simulink model "youbot_predefinedpath_2103"  (R2025b)
settings: Solver=ode3  StartTime=0.0  StopTime=inf  FixedStep=0.01  RelTol=1e-3  EnableMultiTasking=on
values from neighbouring files (symbols this model uses):
  dt = (tf-ti)/n    (= 0.05)    [sss.m]    (also in youbotdynamiceqn.m = 0.1; youbotdynamiceqn_predefinedpath.m)
  Kdx = 1.5    [sss.m]    (also in youbotdynamiceqn_predefinedpath.m)
  Kdy = 1.5    [sss.m]    (also in youbotdynamiceqn_predefinedpath.m)
  Kdz = 0.001    [sss.m]    (also in youbotdynamiceqn_predefinedpath.m = 2.5)
  Kpx = 10    [sss.m]    (also in youbotdynamiceqn_predefinedpath.m = 1.5)
  Kpy = 10    [sss.m]    (also in youbotdynamiceqn_predefinedpath.m = 1.5)
  Kpz = 1    [sss.m]    (also in youbotdynamiceqn_predefinedpath.m = 2.5)
  M_r = [m  0  0 ... (first row only)    [sss.m]    (also in youbotdynamiceqn.m; youbotdynamiceqn_predefinedpath.m)
  M_w = diag([I_w1, I_w2, I_w3, I_w4])    [sss.m]    (also in youbotdynamiceqn.m; youbotdynamiceqn_predefinedpath.m)
  R = (1/r) * [  1, -1, -(L+l) ... (first row only)    [sss.m]    (also in youbotdynamiceqn.m; youbotdynamiceqn_predefinedpath.m)
  R_T = transpose(R)    [sss.m]    (also in youbotdynamiceqn.m; youbotdynamiceqn_predefinedpath.m)
undefined symbols (not defined in the file or in its folder): Angular, Linear
libraries: robotlib x3, robotgazebolib x1, slpidlib x1
settings Model: SimulationMode=accelerator  PacingRate=0.790000  Creator=The MathWorks, Inc.  LastModifiedBy=sinan
settings SolverCC: AlgebraicLoopSolver=TrustRegion  AutoInsertRateTranBlk=on
settings DataIOCC: LimitDataPoints=on  SaveFormat=Array  ReturnWorkspaceOutputs=off
settings OptimizationCC: ZeroExternalMemoryAtStartup=off  ZeroInternalMemoryAtStartup=off  LifeSpan=1  MaxStackSize=64
settings DebuggingCC: AlgebraicLoopMsg=none  SolverPrmCheckMsg=warning  UnconnectedInputMsg=warning  UnconnectedOutputMsg=warning  UnconnectedLineMsg=warning  SFUnexpectedBacktrackingDiag=warning  SFNoUnconditionalDefaultTransitionDiag=warning  SFExecutionAtInitializationDiag=none  ArithmeticOperatorsInVariantConditions=warning
settings HardwareCC: ProdBitPerPointer=32.0  ProdBitPerSizeT=32.0  ProdBitPerPtrDiffT=32.0  ProdLargestAtomicFloat=None  ProdIntDivRoundTo=Undefined  ProdEndianess=Unspecified  ProdWordSize=32.0  ProdHWDeviceType=Generic->Unspecified (assume 32-bit Generic)  TargetHWDeviceType=Generic->Unspecified (assume 32-bit Generic)  UseEmbeddedCoderFeatures=off
settings ModelReferenceCC: EnableRefExpFcnMdlSchedulingChecks=on  PropagateSignalLabelsOutOfModel=off
settings SFSimCC: SimUseLocalCustomCode=off  CustomCodeUndefinedFunction=UseInterfaceOnly  SimTargetLang=C++  SimDLTargetLibrary=mkl-dnn
settings RTWCC: SystemTargetFile=ert.tlc  HardwareBoard=Robot Operating System (ROS)  TLCOptions=-aInlineSetEventsForThisBaseRateFcn=TLC_FALSE -aSuppressMultiTaskScheduler=TLC_FALSE -aRateBasedStepFcn=0  TemplateMakefile=ert_default_tmf  RTWUseLocalCustomCode=off  Toolchain=Catkin  TargetLang=C++  GPUComputeCapability=3.5  Description=Embedded Coder
settings CodeAppCC: StateflowObjectComments=on
settings ERTTargetCC: InlinedParameterPlacement=Hierarchical  RootIOFormat=Structure reference  ConvertIfToSwitch=off  SuppressUnreachableDefaultCases=off  DynamicArrayContainerType=coder::array  MultiwordLength=2048.0  ERTCustomFileBanners=off  CodeInterfacePackaging=C++ class  SupportContinuousTime=on  SupportNonInlinedSFcns=on  RemoveResetFunc=off  SupportVariableSizeSignals=on  ModelStepFunctionPrototypeControlCompliant=off
settings ConfigComp: CovMetricSettings=dw  CovSaveCumulativeToWorkspaceVar=on  CovSaveSingleToWorkspaceVar=on  CovExternalEMLEnable=off  CovSFcnEnable=off
settings SimscapeCC: SimscapeLogDecimation=1  SimscapeLogDataHistory=5000

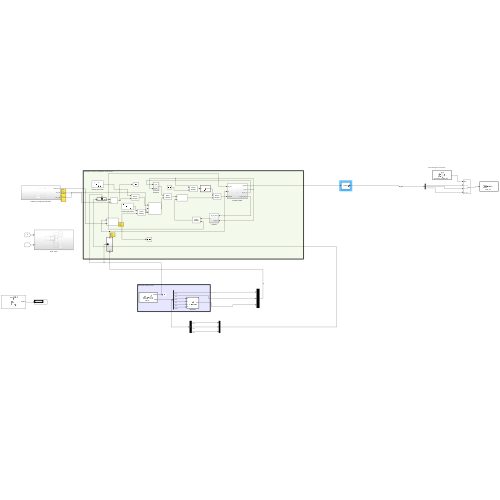
[thumbnail: Simulink's stored preview of the top-level diagram]
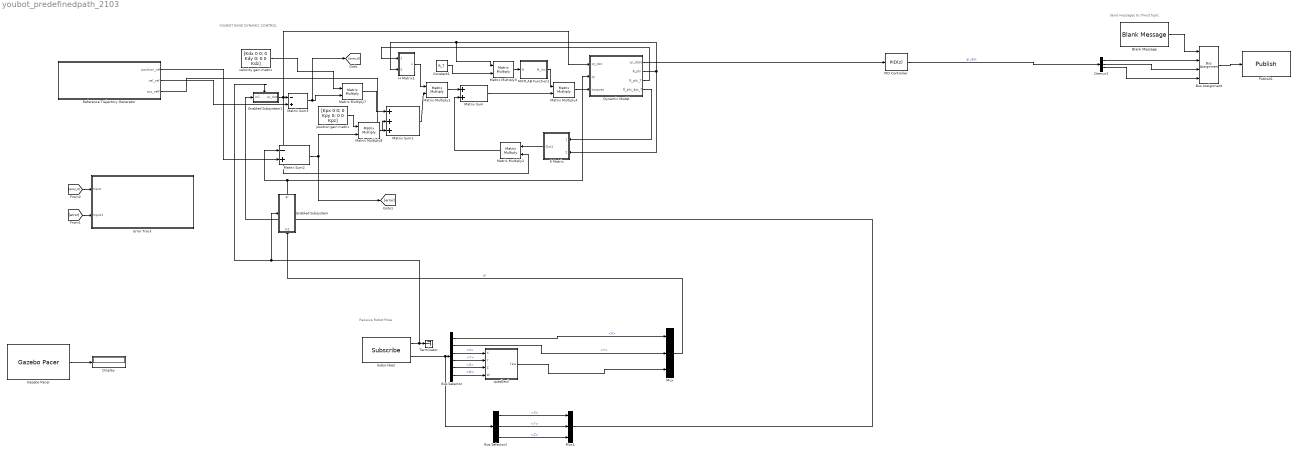
== system youbot_predefinedpath_2103 ==
  note: YOUBOT BASE DYNAMIC CONTROL
  note: Send messages to /Twist topic
  note: Receive Robot Pose
  Blank Message : robotlib/Blank Message  messageClass=Message  entityType=geometry_msgs/Twist  messageType=geometry_msgs/Twist  SampleTime=inf  legacyBusStruct=off
  Bus Assignment : BusAssignment  AssignedSignals=Linear.X,Linear.Y,Angular.Z
  Bus Selector : BusSelector  OutputSignals=Pose.Pose.Position.X,Pose.Pose.Position.Y,Pose.Pose.Orientation.X,Pose.Pose.Orientation.Y,Pose.Pose.Orientation.Z,Pose.Pose.Orientation.W
  Bus Selector1 : BusSelector  OutputSignals=Twist.Twist.Linear.X,Twist.Twist.Linear.Y,Twist.Twist.Angular.Z
  Constant1 : Constant  Value=R_T
  Demux1 : Demux  Outputs=3
  Display : Display
  Dynamic Model : Subsystem
  Enabled Subsystem : Subsystem  TreatAsAtomicUnit=on
  Enabled Subsystem1 : Subsystem  TreatAsAtomicUnit=on
  Error Track : Subsystem
  Gazebo Pacer : robotgazebolib/Gazebo Pacer  ResetBehavior=Reset Gazebo simulation time  SampleTime=0.001
  H Matrix1 : Subsystem
  K Matrix : Subsystem
  MATLAB Function1 : MATLAB Function  TreatAsAtomicUnit=on
  Matrix Sum : Sum
  Matrix Sum1 : Sum  Inputs=+++
  Matrix Sum2 : Sum  Inputs=-+
  Matrix Sum3 : Sum  Inputs=-+
  Matrix Multiply1 : Product  Multiplication=Matrix(*)  SampleTime=dt
  Matrix Multiply{2..4,7..8} (5 alike) : Product  Multiplication=Matrix(*)
  Mux : Mux  Inputs=3
  Mux1 : Mux  Inputs=3
  PID Controller : slpidlib/PID Controller  Controller=PID  Form=Parallel  TimeDomain=Discrete-time  UseExternalTs=off  SampleTime=-1  IntegratorMethod=Forward Euler  FilterMethod=Forward Euler  ControllerParametersSource=internal  P=1  I=0  UseKiTs=off  D=0  UseExternalDerivativeSource=off  N=100  UseFilter=on  TunerSelectOption=Transfer Function Based (PID Tuner App)  InitialConditionSource=internal  InitialConditionForIntegrator=0  InitialConditionForFilter=0  DifferentiatorICPrevScaledInput=0  ExternalReset=none  TrackingMode=off  Kt=1  LimitOutput=on  SatLimitsSource=internal  UpperSaturationLimit=1.5  LowerSaturationLimit=-1.5  LinearizeAsGain=on  AntiWindupMode=clamping  Kb=1  LimitIntegrator=off  UpperIntegratorSaturationLimit=inf  LowerIntegratorSaturationLimit=-inf  POutMin=[]  POutMax=[]  IOutMin=[]  IOutMax=[]  DOutMin=[]  DOutMax=[]  NOutMin=[]  NOutMax=[]  SumOutMin=[]  SumOutMax=[]  SaturationOutMin=[]  SaturationOutMax=[]  PParamMin=[]  PParamMax=[]  IParamMin=[]  IParamMax=[]  DParamMin=[]  DParamMax=[]  NParamMin=[]  NParamMax=[]  KbParamMin=[]  KbParamMax=[]  KtParamMin=[]  KtParamMax=[]  KbOutMin=[]  KbOutMax=[]  KtOutMin=[]  KtOutMax=[]  IntegratorOutMin=[]  IntegratorOutMax=[]  FilterOutMin=[]  FilterOutMax=[]  SumI1OutMin=[]  SumI1OutMax=[]  SumI2OutMin=[]  SumI2OutMax=[]  SumI3OutMin=[]  SumI3OutMax=[]  SumI4OutMin=[]  SumI4OutMax=[]  SumDOutMin=[]  SumDOutMax=[]  DifferentiatorOutMin=[]  DifferentiatorOutMax=[]  FilterDiffOutCoefMin=[]  FilterDiffOutCoefMax=[]  ReciprocalOutMin=[]  ReciprocalOutMax=[]  SumDenOutMin=[]  SumDenOutMax=[]  SumNumOutMin=[]  SumNumOutMax=[]  DivideOutMin=[]  DivideOutMax=[]  UdiffTsProdOutMin=[]  UdiffTsProdOutMax=[]  NTsProdOutMin=[]  NTsProdOutMax=[]  UintegralTsProdOutMin=[]  UintegralTsProdOutMax=[]  UngainTsProdOutMin=[]  UngainTsProdOutMax=[]  ClampingZeroOutDataTypeStr=Inherit: Inherit via back propagation  ClampingZeroOutMin=[]  ClampingZeroOutMax=[]  FilterDenConstantOutDataTypeStr=Inherit: Inherit via back propagation  FilterDenConstantOutMin=[]  FilterDenConstantOutMax=[]  PCopyOutDataTypeStr=Inherit: Inherit via back propagation  PCopyOutMin=[]  PCopyOutMax=[]  NCopyOutDataTypeStr=Inherit: Inherit via back propagation  NCopyOutMin=[]  NCopyOutMax=[]  IntegratorContinuousStateAttributes=''  IntegratorStateMustResolveToSignalObject=off  IntegratorRTWStateStorageClass=Auto  FilterContinuousStateAttributes=''  FilterStateMustResolveToSignalObject=off  FilterRTWStateStorageClass=Auto  ParallelPVariant=InternalParameters  IdealPVariant=Disabled  IVariant=InternalParameters  DVariant=InternalParameters  IntegratorVariant=Discrete  SatVariant=Enabled  AWVariant=DiscClampingParallel  PCopyVariant=Disabled  TRVariant=Disabled  FdbkBlocksVariant=Forward  IdealPFdbkVariant=Disabled  SatFdbkVariant=Disabled  DerivativeFilterVariant=ForwardEulerFilter  NVariant=InternalParameters  NCopyVariant=Disabled  FilterICVariant=InternalICsFilter  IntegratorICVariant=InternalICs  ExternalResetVariant=Disabled  TRSumVariant=Passthrough  SumFdbkVariant=Disabled  SumVariant=Sum_PID  TsampFilterVariant=InternalTs  TsampNgainVariant=Passthrough  TsampIntegralVariant=Disabled_SignalSpec  ExternalSaturationOutDataTypeStr=Inherit: Same as second input  DerivativeSourceVariant=ErrorSignal  PreIntVariant=InternalPreInt
  Publish1 : robotlib/Publish  topicSource=Select from ROS network  topic=/cmd_vel  messageType=geometry_msgs/Twist  legacyBusStruct=off  messageQueueLength=105
  Reference Trajectory Generator : Subsystem
  Subscribe2 : robotlib/Subscribe  topicSource=Select from ROS network  topic=/odom  messageType=nav_msgs/Odometry  SampleTime=-1  legacyBusStruct=off  messageQueueLength=1
  Terminator : Terminator
  position gain matrix : Constant  Value=[Kpx 0 0; 0 Kpy 0; 0 0 Kpz]
  quad2eul : MATLAB Function  TreatAsAtomicUnit=on
  velocity gain matrix : Constant  Value=[Kdx 0 0; 0 Kdy 0; 0 0 Kdz]
  wires:
  Dynamic Model/1(qr_ddot) -> PID Controller/1
  Matrix Multiply4/1 -> Dynamic Model/3(torques)
  Matrix Multiply2/1 -> Matrix Sum/2
  K Matrix/1(Out1) -> Matrix Multiply2/1
  Matrix Multiply7/1 -> Matrix Sum1/1
  Matrix Multiply3/1 -> MATLAB Function1/1(N)
  Matrix Sum1/1 -> Matrix Multiply1/2
  H Matrix1/1(Out1) -> Matrix Multiply1/1
  Constant1/1 -> Matrix Multiply3/2
  Dynamic Model/4(R_phi_dot_T) -> K Matrix/1(R_phi_dot_T)
  MATLAB Function1/1(N_inv) -> Matrix Multiply4/1
  Dynamic Model/3(R_phi_T) -> H Matrix1/1(R_phi_T)
  Matrix Sum3/1 -> Matrix Multiply7/2, [error_d]
  PID Controller/1 -> Demux1/1  "qr_dot"
  Matrix Sum2/1 -> [error], Matrix Multiply8/2
  position gain matrix/1 -> Matrix Multiply8/1
  Dynamic Model/2(R_phi) -> K Matrix/2(R_phi_T), Matrix Multiply3/1, H Matrix1/2(R_phi)
  Matrix Multiply1/1 -> Matrix Sum/1
  Matrix Sum/1 -> Matrix Multiply4/2
  Matrix Multiply8/1 -> Matrix Sum1/2
  velocity gain matrix/1 -> Matrix Multiply7/1
  Reference Trajectory Generator/1(position_ref) -> Matrix Sum2/2
  Reference Trajectory Generator/3(acc_reff) -> Matrix Sum1/3
  [error] -> Error Track/2(Input1)
  [error_d] -> Error Track/1(Input)
  Demux1/3 -> Bus Assignment/4
  Demux1/2 -> Bus Assignment/3
  Bus Assignment/1 -> Publish1/1
  Blank Message/1 -> Bus Assignment/1
  Demux1/1 -> Bus Assignment/2
  Bus Selector/2 -> Mux/2  "<Y>"
  Bus Selector/3 -> quad2eul/1(X)  "<X>"
  quad2eul/1(Yaw) -> Mux/3
  Bus Selector/1 -> Mux/1  "<X>"
  Bus Selector/5 -> quad2eul/3(Z)  "<Z>"
  Subscribe2/2 -> Bus Selector1/1, Bus Selector/1
  Bus Selector/6 -> quad2eul/4(W)  "<W>"
  Subscribe2/1 -> Enabled Subsystem1/Enable, Enabled Subsystem/Enable, Terminator/1
  Bus Selector/4 -> quad2eul/2(Y)  "<Y>"
  Enabled Subsystem/1(qr) -> Dynamic Model/2(qr), Matrix Sum2/1
  Bus Selector1/1 -> Mux1/1  "<X>"
  Bus Selector1/2 -> Mux1/2  "<Y>"
  Bus Selector1/3 -> Mux1/3  "<Z>"
  Enabled Subsystem1/1(qr_dot) -> Dynamic Model/1(qr_dot), Matrix Sum3/1, Matrix Multiply2/2
  Mux1/1 -> Enabled Subsystem1/1(In1)
  Mux/1 -> Enabled Subsystem/1(In1)  "qr"
  Reference Trajectory Generator/2(vel_ref) -> Matrix Sum3/2
  Gazebo Pacer/1 -> Display/1

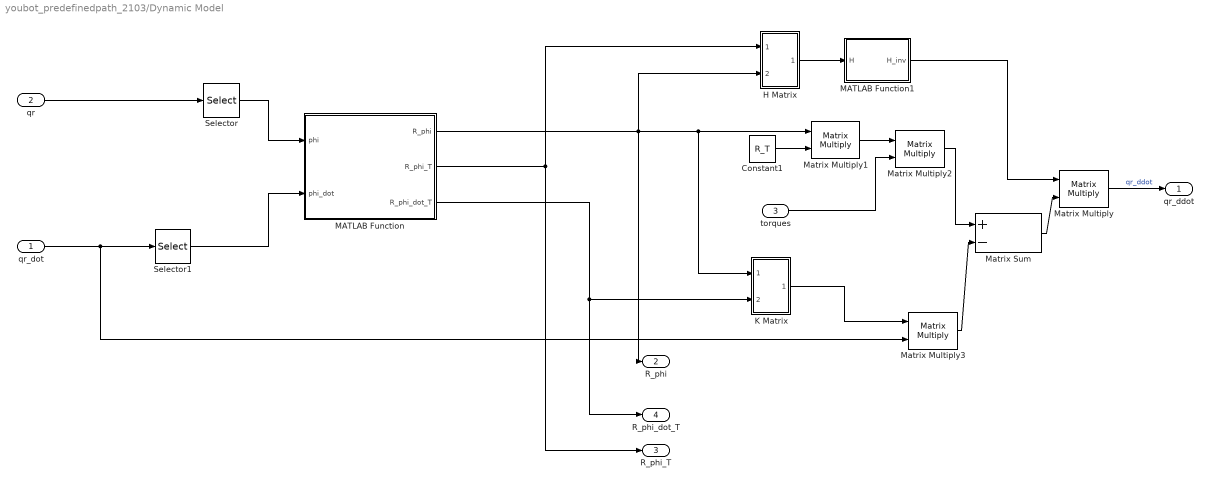
== system youbot_predefinedpath_2103/Dynamic Model ==
  qr_dot : Inport
  qr : Inport  Port=2
  torques : Inport  Port=3
  Constant1 : Constant  Value=R_T
  H Matrix : Subsystem
  K Matrix : Subsystem
  MATLAB Function : MATLAB Function  TreatAsAtomicUnit=on
  MATLAB Function1 : MATLAB Function  TreatAsAtomicUnit=on
  Matrix Sum : Sum  Inputs=+-
  Matrix Multiply{,1..3} (4 alike) : Product  Multiplication=Matrix(*)
  Selector : Selector  InputPortWidth=3  IndexOptions=Index vector (dialog)  Indices=[3]  OutputSizes=1
  Selector1 : Selector  InputPortWidth=3  IndexOptions=Index vector (dialog)  Indices=[3]  OutputSizes=1
  qr_ddot : Outport  PortDimensions=[3 1]
  R_phi : Outport  Port=2
  R_phi_T : Outport  Port=3
  R_phi_dot_T : Outport  Port=4
  wires:
  torques/1 -> Matrix Multiply2/2
  MATLAB Function/3(R_phi_dot_T) -> R_phi_dot_T/1, K Matrix/2(R_phi_dot_T)
  MATLAB Function/2(R_phi_T) -> R_phi_T/1, H Matrix/1(In2)
  Matrix Multiply2/1 -> Matrix Sum/1
  Matrix Multiply3/1 -> Matrix Sum/2
  K Matrix/1(Out1) -> Matrix Multiply3/1
  MATLAB Function1/1(H_inv) -> Matrix Multiply/1
  MATLAB Function/1(R_phi) -> K Matrix/1(R_phi), Matrix Multiply1/1, R_phi/1, H Matrix/2(In1)
  Constant1/1 -> Matrix Multiply1/2
  Matrix Multiply1/1 -> Matrix Multiply2/1
  Matrix Multiply/1 -> qr_ddot/1  "qr_ddot"
  Matrix Sum/1 -> Matrix Multiply/2
  H Matrix/1(Out1) -> MATLAB Function1/1(H)
  Selector/1 -> MATLAB Function/1(phi)
  Selector1/1 -> MATLAB Function/2(phi_dot)
  qr/1 -> Selector/1
  qr_dot/1 -> Matrix Multiply3/2, Selector1/1

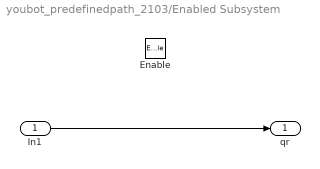
== system youbot_predefinedpath_2103/Enabled Subsystem ==
  In1 : Inport
  Enable : EnablePort
  qr : Outport
  wires:
  In1/1 -> qr/1

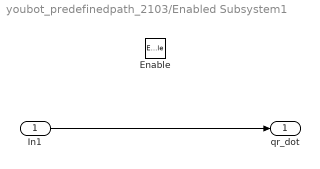
== system youbot_predefinedpath_2103/Enabled Subsystem1 ==
  In1 : Inport
  Enable : EnablePort
  qr_dot : Outport
  wires:
  In1/1 -> qr_dot/1

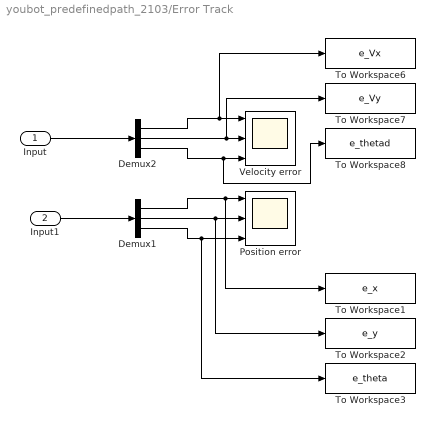
== system youbot_predefinedpath_2103/Error Track ==
  Input : Inport
  Input1 : Inport  Port=2
  Demux1 : Demux  Outputs=3
  Demux2 : Demux  Outputs=3
  Position error : Scope  NumInputPorts=3
      settings: ActiveDisplayYMinimum=-0.37573  ActiveDisplayYMaximum=1.28023  DataLoggingVariableName=ScopeData2
  To Workspace1 : ToWorkspace  VariableName=e_x  SaveFormat=Timeseries  SampleTime=-1
  To Workspace2 : ToWorkspace  VariableName=e_y  SaveFormat=Timeseries  SampleTime=-1
  To Workspace3 : ToWorkspace  VariableName=e_theta  SaveFormat=Timeseries  SampleTime=-1
  To Workspace6 : ToWorkspace  VariableName=e_Vx  SaveFormat=Timeseries  SampleTime=-1
  To Workspace7 : ToWorkspace  VariableName=e_Vy  SaveFormat=Timeseries  SampleTime=-1
  To Workspace8 : ToWorkspace  VariableName=e_thetad  SaveFormat=Timeseries  SampleTime=-1
  Velocity error : Scope  NumInputPorts=3
      settings: ActiveDisplayYMinimum=0.240186  ActiveDisplayYMaximum=0.24023
  wires:
  Input1/1 -> Demux1/1
  Demux2/3 -> To Workspace8/1, Velocity error/3
  Demux1/1 -> To Workspace1/1, Position error/1
  Input/1 -> Demux2/1
  Demux1/2 -> To Workspace2/1, Position error/2
  Demux2/2 -> To Workspace7/1, Velocity error/2
  Demux1/3 -> To Workspace3/1, Position error/3
  Demux2/1 -> To Workspace6/1, Velocity error/1

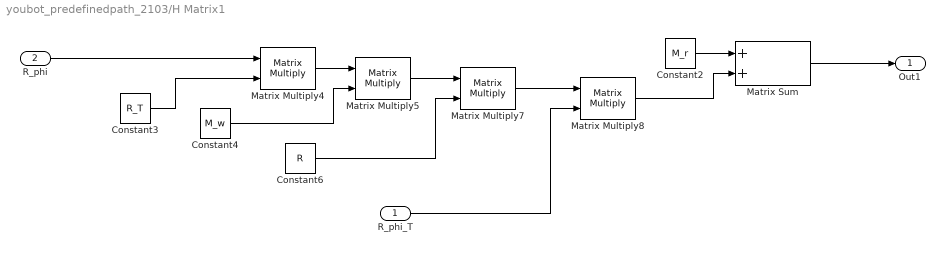
== system youbot_predefinedpath_2103/H Matrix1 ==
  R_phi_T : Inport
  R_phi : Inport  Port=2
  Constant2 : Constant  Value=M_r
  Constant3 : Constant  Value=R_T
  Constant4 : Constant  Value=M_w
  Constant6 : Constant  Value=R
  Matrix Sum : Sum
  Matrix Multiply{4..5,7..8} (4 alike) : Product  Multiplication=Matrix(*)  SampleTime=dt
  Out1 : Outport
  wires:
  Constant2/1 -> Matrix Sum/1
  Matrix Multiply4/1 -> Matrix Multiply5/1
  R_phi_T/1 -> Matrix Multiply8/2
  Matrix Multiply7/1 -> Matrix Multiply8/1
  Constant6/1 -> Matrix Multiply7/2
  Matrix Multiply8/1 -> Matrix Sum/2
  Constant4/1 -> Matrix Multiply5/2
  Constant3/1 -> Matrix Multiply4/2
  Matrix Sum/1 -> Out1/1
  Matrix Multiply5/1 -> Matrix Multiply7/1
  R_phi/1 -> Matrix Multiply4/1

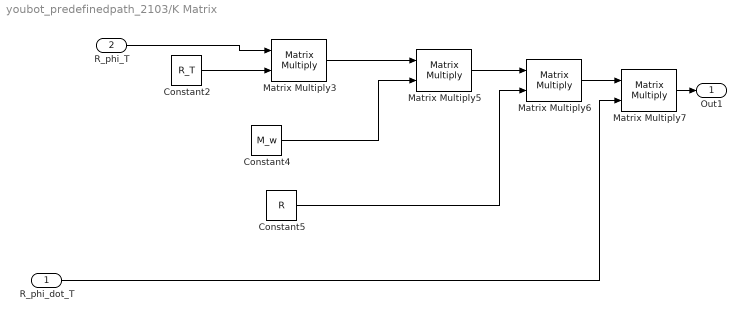
== system youbot_predefinedpath_2103/K Matrix ==
  R_phi_dot_T : Inport
  R_phi_T : Inport  Port=2
  Constant2 : Constant  Value=R_T
  Constant4 : Constant  Value=M_w
  Constant5 : Constant  Value=R
  Matrix Multiply{3,5..7} (4 alike) : Product  Multiplication=Matrix(*)
  Out1 : Outport  PortDimensions=[3 3]
  wires:
  Matrix Multiply7/1 -> Out1/1
  Matrix Multiply6/1 -> Matrix Multiply7/1
  Matrix Multiply3/1 -> Matrix Multiply5/1
  R_phi_T/1 -> Matrix Multiply3/1
  Constant4/1 -> Matrix Multiply5/2
  Constant5/1 -> Matrix Multiply6/2
  R_phi_dot_T/1 -> Matrix Multiply7/2
  Constant2/1 -> Matrix Multiply3/2
  Matrix Multiply5/1 -> Matrix Multiply6/1

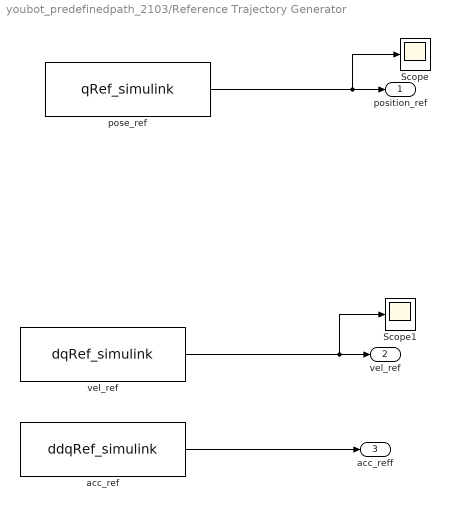
== system youbot_predefinedpath_2103/Reference Trajectory Generator ==
  " vel_ref" : FromWorkspace  VariableName=dqRef_simulink
  Scope : Scope
      settings: ActiveDisplayYMinimum=-5.00483  ActiveDisplayYMaximum=2.55609
  Scope1 : Scope
      settings: ActiveDisplayYMinimum=-1  ActiveDisplayYMaximum=1  DataLoggingVariableName=ScopeData2
  acc_ref : FromWorkspace  VariableName=ddqRef_simulink
  pose_ref : FromWorkspace  VariableName=qRef_simulink
  position_ref : Outport
  vel_ref : Outport  Port=2
  acc_reff : Outport  Port=3
  wires:
  acc_ref/1 -> acc_reff/1
  pose_ref/1 -> Scope/1, position_ref/1
  " vel_ref"/1 -> Scope1/1, vel_ref/1

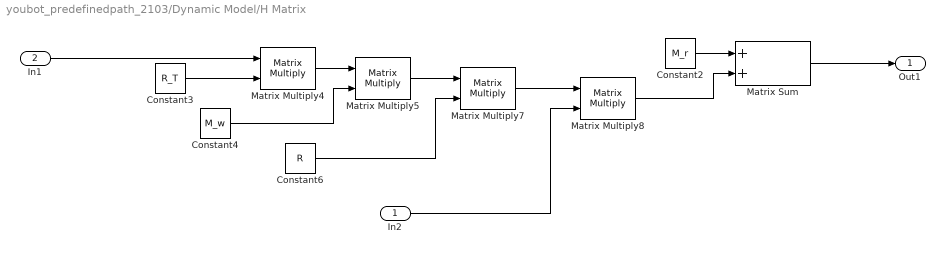
== system youbot_predefinedpath_2103/Dynamic Model/H Matrix ==
  In2 : Inport
  In1 : Inport  Port=2
  Constant2 : Constant  Value=M_r
  Constant3 : Constant  Value=R_T
  Constant4 : Constant  Value=M_w
  Constant6 : Constant  Value=R
  Matrix Sum : Sum
  Matrix Multiply{4..5,7..8} (4 alike) : Product  Multiplication=Matrix(*)
  Out1 : Outport
  wires:
  In1/1 -> Matrix Multiply4/1
  Matrix Multiply5/1 -> Matrix Multiply7/1
  Matrix Sum/1 -> Out1/1
  Constant3/1 -> Matrix Multiply4/2
  Constant4/1 -> Matrix Multiply5/2
  Matrix Multiply8/1 -> Matrix Sum/2
  Constant6/1 -> Matrix Multiply7/2
  Matrix Multiply7/1 -> Matrix Multiply8/1
  In2/1 -> Matrix Multiply8/2
  Matrix Multiply4/1 -> Matrix Multiply5/1
  Constant2/1 -> Matrix Sum/1

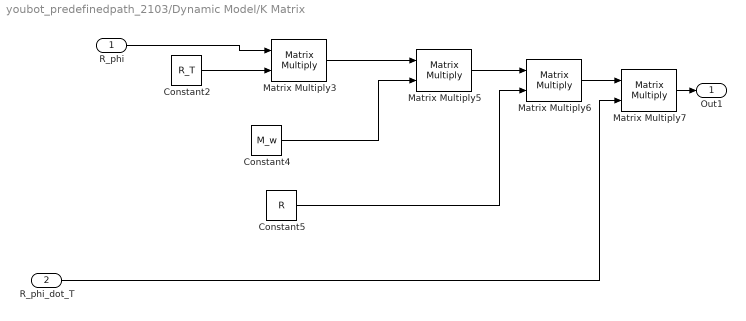
== system youbot_predefinedpath_2103/Dynamic Model/K Matrix ==
  R_phi : Inport
  R_phi_dot_T : Inport  Port=2
  Constant2 : Constant  Value=R_T
  Constant4 : Constant  Value=M_w
  Constant5 : Constant  Value=R
  Matrix Multiply{3,5..7} (4 alike) : Product  Multiplication=Matrix(*)
  Out1 : Outport
  wires:
  Matrix Multiply7/1 -> Out1/1
  Matrix Multiply6/1 -> Matrix Multiply7/1
  Matrix Multiply3/1 -> Matrix Multiply5/1
  R_phi/1 -> Matrix Multiply3/1
  Constant4/1 -> Matrix Multiply5/2
  Constant5/1 -> Matrix Multiply6/2
  R_phi_dot_T/1 -> Matrix Multiply7/2
  Constant2/1 -> Matrix Multiply3/2
  Matrix Multiply5/1 -> Matrix Multiply6/1

== matlab function youbot_predefinedpath_2103/Dynamic Model/MATLAB Function1 ==
  data: H input; H_inv output
function H_inv = fcn(H)

H_inv = inv(H);

== matlab function youbot_predefinedpath_2103/Dynamic Model/MATLAB Function ==
  data: phi input; R_phi output size=[3 3]; phi_dot input; R_phi_T output size=[3 3]; R_phi_dot_T output size=[3 3]
function [R_phi, R_phi_T, R_phi_dot_T] = fcn(phi, phi_dot)

    % Giriş değerlerini göster
    fprintf('phi: %f\n', phi);
    fprintf('phi_dot: %f\n', phi_dot);

    % NaN kontrolü
    if isnan(phi)
        warning('phi is NaN');
    end
    if isnan(phi_dot)
        warning('phi_dot is NaN');
    end

    R_phi = [ cos(phi), -sin(phi), 0;
              sin(phi),  cos(phi), 0;
                    0  ,        0 , 1];

    R_phi_dot = [ -sin(phi)*phi_dot, -cos(phi)*phi_dot, 0;
                   cos(phi)*phi_dot,  -sin(phi)*phi_dot, 0;
                             0      ,              0    , 0];

    % R_phi_dot matrisindeki NaN'leri kontrol et
    if any(isnan(R_phi_dot), 'all')
        warning('R_phi_dot contains NaN values');
        disp('R_phi_dot matrix:');
        disp(R_phi_dot);
    end
   if isnan(phi) || isnan(phi_dot)
    disp('phi or phi_dot is NaN at this timestep!');
    disp(sprintf('phi = %f', phi));
    disp(sprintf('phi_dot = %f', phi_dot));
    end
    R_phi_T = transpose(R_phi);
    R_phi_dot_T = transpose(R_phi_dot);

    % Sonuçları göster
    disp('R_phi_dot_T:');
    disp(R_phi_dot_T);

end

== matlab function youbot_predefinedpath_2103/MATLAB Function1 ==
  data: N input; N_inv output
function N_inv = fcn(N)

N_inv = pinv(N);

== matlab function youbot_predefinedpath_2103/quad2eul ==
  data: X input; Yaw output; Y input; Z input; W input
function Yaw = quat2eulBlk(X, Y, Z, W)
%#codegen
% Quaternion'dan [0, 2pi] aralığında yaw açısını çıkarır.

% Euler açılarını elde et (varsayılan dönüşüm sırası: ZYX → [yaw, pitch, roll])
eulerAngles = quat2eul([W, X, Y, Z]);  % [yaw, pitch, roll], yaw ∈ [-pi, pi]

% Yaw açısını [0, 2pi] aralığına çevir
Yaw = eulerAngles(1);
end
